simulink model "sgMdl_IO581_Loopback"  (R2024b)
settings: Solver=FixedStepAuto  StartTime=0.0  StopTime=inf  RelTol=1e-3  EnableMultiTasking=on
undefined symbols (not defined in the file): standard
libraries: speedgoatlib_serial x5, slrealtimeseriallib x4, simulink x1
Description:
  | IO581 - Loopback
settings Model: ModifiedByFormat=Speedgoat  Creator=Speedgoat  LastModifiedBy=Speedgoat
settings SolverCC: ConcurrentTasks=on  AlgebraicLoopSolver=TrustRegion  PositivePriorityOrder=on  InsertRTBMode=Never (minimum delay)
settings DataIOCC: LimitDataPoints=on  SaveFormat=Array  SignalLoggingSaveFormat=ModelDataLogs  ReturnWorkspaceOutputs=off
settings OptimizationCC: BlockReduction=off  OptimizeBlockIOStorage=off  BufferReuse=off  GlobalBufferReuse=off  ExpressionFolding=off  ExpressionDepthLimit=2147483647  LocalBlockOutputs=off  OptimizeDataStoreBuffers=off  BusAssignmentInplaceUpdate=off
settings DebuggingCC: UnderspecifiedInitializationDetection=Classic  MergeDetectMultiDrivingBlocksExec=none  SolverPrmCheckMsg=warning  TasksWithSamePriorityMsg=none  FcnCallInpInsideContextMsg=warning  StateNameClashWarn=warning  SFUnexpectedBacktrackingDiag=warning  SFNoUnconditionalDefaultTransitionDiag=warning  SFExecutionAtInitializationDiag=none  ArithmeticOperatorsInVariantConditions=warning
settings HardwareCC: ProdBitPerLong=64  ProdLongLongMode=on  ProdHWDeviceType=Intel->x86-64 (Linux 64)
settings ModelReferenceCC: EnableRefExpFcnMdlSchedulingChecks=on  PropagateSignalLabelsOutOfModel=off
settings SFSimCC: SimUseLocalCustomCode=off  CustomCodeUndefinedFunction=UseInterfaceOnly
settings RTWCC: Description=Speedgoat Real-Time Target Machine  SystemTargetFile=speedgoat.tlc  TemplateMakefile=slrealtime_default_tmf  RTWUseLocalCustomCode=off  Toolchain=Simulink Real-Time Toolchain  BuildConfiguration=Faster Runs  TargetLang=C++  GPUComputeCapability=3.5  DLArmComputeVersion=19.05
settings CodeAppCC: StateflowObjectComments=on
settings SimulinkRealTimeTargetCC: SubcomponentCodeInterfacePackaging=Reusable function  InstructionSetFMA=off  LogToMDFFile=off  SLRTFileLogMaxRuns=10  UseGCCFastMath=on
settings ConfigComp: CovMetricSettings=dw  CovSaveCumulativeToWorkspaceVar=on  CovSaveSingleToWorkspaceVar=on  CovExternalEMLEnable=off  CovSFcnEnable=off  CovBoundaryAbsTol=1.0e-5

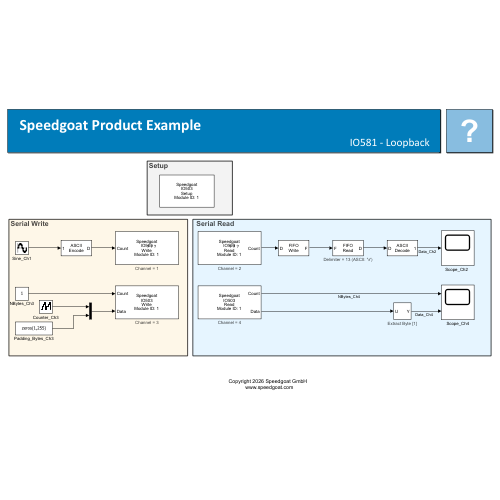
[thumbnail: Simulink's stored preview of the top-level diagram]
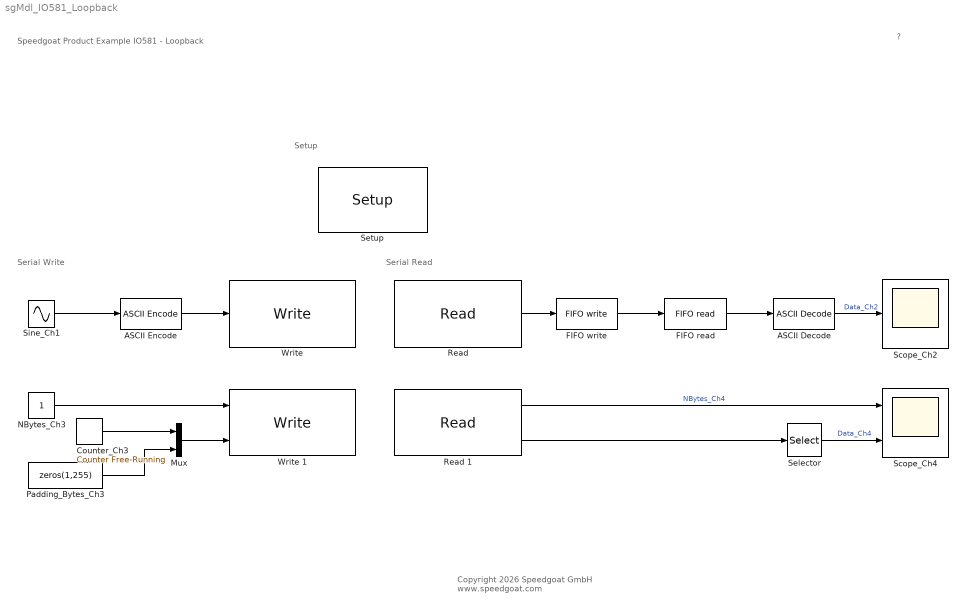
== system sgMdl_IO581_Loopback ==
  note: Setup
  note: Serial Write
  note: Serial Read
  note: Speedgoat Product Example
      | IO581 - Loopback
  note: ?
  note: Copyright 2026 Speedgoat GmbH
      |  www.speedgoat.com
  ASCII Decode : slrealtimeseriallib/ASCII Decode  format=%f\r  nvars=1  vartypes={'double'}
  ASCII Encode : slrealtimeseriallib/ASCII Encode  format=%f\r  nvars=1  maxlength=256  vartypes={ 'double' }
  Counter_Ch3 : simulink/Sources/Counter Free-Running  NumBits=8  tsamp=0.01
  FIFO read : slrealtimeseriallib/FIFO read  maxsize=2*256  minsize=1  usedelimiter=on  delimiter=13  outputtype=8 bit uint null terminated  enable=off  enableout=off  sampletime=0.01
      settings: AttributesFormatString=Delimiter = %<delimiter> (ASCII: '\r')
  FIFO write : slrealtimeseriallib/FIFO write  size=128  inputtype=8 bit uint null terminated  present=off  sampletime=-1  id=Rx Ch2 overflow
  Mux : Mux  Inputs=2
  NBytes_Ch3 : Constant  OutDataTypeStr=Inherit: Inherit via back propagation  SampleTime=0.01
  Padding_Bytes_Ch3 : Constant  Value=zeros(1,255)  OutDataTypeStr=Inherit: Inherit via back propagation  SampleTime=0.01
  "Read " : speedgoatlib_serial/Speedgoat Shared blocks/Read   parModuleType=IO581  parModuleId=1  parChannel=2  parSampleTime=0.01  parFlush=on  parEnLegacy=on  parDataType=8 bit uint null terminated  parSlot=-1  parRxSwFifoSize=256
      settings: AttributesFormatString=Channel = %<parChannel>
  Read 1 : speedgoatlib_serial/Speedgoat Shared blocks/Read   parModuleType=IO581  parModuleId=1  parChannel=4  parSampleTime=0.01  parFlush=on  parEnLegacy=off  parDataType=count+32 bit uint  parSlot=-1  parRxSwFifoSize=256
      settings: AttributesFormatString=Channel = %<parChannel>
  "Scope_Ch2  " : Scope
  Scope_Ch4 : Scope  NumInputPorts=2
  Selector : Selector  IndexOptions=Index vector (dialog)  Indices=[1]  OutputSizes=1
      settings: AttributesFormatString=Extract Byte %<Indices>
  "Setup " : speedgoatlib_serial/Speedgoat Shared blocks/Setup   parModuleType=IO581  parModuleId=1  parSlot=-1  parOscillator=44.2368  parOscillator581=125  parTransceiver1=RS232  parTransceiver2=RS232  parTransceiver3=RS232  parTransceiver4=RS232  parTransceiver5=RS232  parTransceiver6=RS232  parTransceiver7=RS232  parTransceiver8=RS232  parTxTerm1=off  parRxTerm1=off  parMessageMonitoring1=off  parAutoTurnaround1=off  parTurnaroundDelay1=0  parStandardBaud1=on  parBaudrate1=921600  parBaudDivisor1=1  parSamplingRate1=16x (standard)  parPrescale1=None  parCalcBaud1=7812500  parParity1=None  parDataBits1=8  parStopBits1=1  parTxTrigLvl1=1  parRxTrigLvl1=8  parHandshake1=none  parRtsHysteresis1=0  parXon1=17  parXoff1=19  parTxSwFifoSize1=256  parRxSwFifoSize1=256  parTxTerm2=off  parRxTerm2=off  parMessageMonitoring2=off  parAutoTurnaround2=off  parTurnaroundDelay2=0  parStandardBaud2=on  parBaudrate2=921600  parBaudDivisor2=1  parSamplingRate2=16x (standard)  parPrescale2=None  parCalcBaud2=7812500  parParity2=None  parDataBits2=8  parStopBits2=1  parTxTrigLvl2=1  parRxTrigLvl2=8  parHandshake2=none  parRtsHysteresis2=0  parXon2=17  parXoff2=19  parTxSwFifoSize2=256  parRxSwFifoSize2=256  parTxTerm3=off  parRxTerm3=off  parMessageMonitoring3=off  parAutoTurnaround3=off  parTurnaroundDelay3=0  parStandardBaud3=on  parBaudrate3=921600  parBaudDivisor3=1  parSamplingRate3=16x (standard)  parPrescale3=None  parCalcBaud3=7812500  parParity3=None  parDataBits3=8  parStopBits3=1  parTxTrigLvl3=1  parRxTrigLvl3=8  parHandshake3=none  parRtsHysteresis3=0  parXon3=17  parXoff3=19  parTxSwFifoSize3=256  parRxSwFifoSize3=256  parTxTerm4=off  parRxTerm4=off  parMessageMonitoring4=off  parAutoTurnaround4=off  parTurnaroundDelay4=0  parStandardBaud4=on  parBaudrate4=921600  parBaudDivisor4=1  parSamplingRate4=16x (standard)  parPrescale4=None  parCalcBaud4=7812500  parParity4=None  parDataBits4=8  parStopBits4=1  parTxTrigLvl4=1  parRxTrigLvl4=8  parHandshake4=none  parRtsHysteresis4=0  parXon4=17  parXoff4=19  parTxSwFifoSize4=256  parRxSwFifoSize4=256  parTxTerm5=off  parRxTerm5=off  parMessageMonitoring5=off  parAutoTurnaround5=off  parTurnaroundDelay5=0  parStandardBaud5=on  parBaudrate5=115200  parBaudDivisor5=1  parSamplingRate5=16x (standard)  parPrescale5=None  parCalcBaud5=2764800  parParity5=None  parDataBits5=8  parStopBits5=1  parTxTrigLvl5=1  parRxTrigLvl5=1  parHandshake5=none  parRtsHysteresis5=0  parXon5=17  parXoff5=19  parTxSwFifoSize5=1024  parRxSwFifoSize5=1024  parTxTerm6=off  parRxTerm6=off  parMessageMonitoring6=off  parAutoTurnaround6=off  parTurnaroundDelay6=0  parStandardBaud6=on  parBaudrate6=115200  parBaudDivisor6=1  parSamplingRate6=16x (standard)  parPrescale6=None  parCalcBaud6=2764800  parParity6=None  parDataBits6=8  parStopBits6=1  parTxTrigLvl6=1  parRxTrigLvl6=1  parHandshake6=none  parRtsHysteresis6=0  parXon6=17  parXoff6=19  parTxSwFifoSize6=1024  parRxSwFifoSize6=1024  parTxTerm7=off  parRxTerm7=off  parMessageMonitoring7=off  parAutoTurnaround7=off  parTurnaroundDelay7=0  parStandardBaud7=on  parBaudrate7=115200  parBaudDivisor7=1  parSamplingRate7=16x (standard)  parPrescale7=None  parCalcBaud7=2764800  parParity7=None  parDataBits7=8  parStopBits7=1  parTxTrigLvl7=1  parRxTrigLvl7=1  parHandshake7=none  parRtsHysteresis7=0  parXon7=17  parXoff7=19  parTxSwFifoSize7=1024  parRxSwFifoSize7=1024  parTxTerm8=off  parRxTerm8=off  parMessageMonitoring8=off  parAutoTurnaround8=off  parTurnaroundDelay8=0  parStandardBaud8=on  parBaudrate8=115200  parBaudDivisor8=1  parSamplingRate8=16x (standard)  parPrescale8=None  parCalcBaud8=2764800  parParity8=None  parDataBits8=8  parStopBits8=1  parTxTrigLvl8=1  parRxTrigLvl8=1  parHandshake8=none  parRtsHysteresis8=0  parXon8=17  parXoff8=19  parTxSwFifoSize8=1024  parRxSwFifoSize8=1024
      settings: SourceProductName=Simulink Real-Time: Speedgoat I/O Driver Library
  Sine_Ch1 : Sin  Amplitude=10  Bias=127  Frequency=1*2*pi  SampleTime=0.01
  "Write " : speedgoatlib_serial/Speedgoat Shared blocks/Write   parModuleType=IO581  parModuleId=1  parChannel=1  parSampleTime=-1  parEnLegacy=on  parDataType=8 bit uint null terminated  parMdlStopMsgEnable=off  parMdlStopMsgData=['CONF' char(13)]  parMdlStopFifoOptions=Write to TX FIFO directly  parMdlStopMsgsDataArr=[67 79 78 70 13]  parMdlStopMsgsDataSize=5  parSlot=-1  parTxSwFifoSize=256
      settings: AttributesFormatString=Channel = %<parChannel>
  Write 1 : speedgoatlib_serial/Speedgoat Shared blocks/Write   parModuleType=IO581  parModuleId=1  parChannel=3  parSampleTime=-1  parEnLegacy=off  parDataType=8 bit uint null terminated  parMdlStopMsgEnable=off  parMdlStopMsgData=['CONF' char(13)]  parMdlStopFifoOptions=Write to TX FIFO directly  parMdlStopMsgsDataArr=[67 79 78 70 13]  parMdlStopMsgsDataSize=5  parSlot=-1  parTxSwFifoSize=256
      settings: AttributesFormatString=Channel = %<parChannel>
  wires:
  Sine_Ch1/1 -> ASCII Encode/1
  ASCII Decode/1 -> "Scope_Ch2  "/1  "Data_Ch2"
  FIFO write/1 -> FIFO read/1
  "Read "/1 -> FIFO write/1
  ASCII Encode/1 -> "Write "/1
  FIFO read/1 -> ASCII Decode/1
  NBytes_Ch3/1 -> Write 1/1
  Read 1/1 -> Scope_Ch4/1  "NBytes_Ch4"
  Read 1/2 -> Selector/1
  Mux/1 -> Write 1/2
  Counter_Ch3/1 -> Mux/1
  Padding_Bytes_Ch3/1 -> Mux/2
  Selector/1 -> Scope_Ch4/2  "Data_Ch4"
